simulink model "pto10Melo"  (R2021a)
settings: Solver=VariableStepAuto  StartTime=0.0  StopTime=10.0  RelTol=1e-3
values from neighbouring files (symbols this model uses):
  k = acker(A_aux, B_aux, p)    [Posibletaller3.m]
  L = acker(A', C', P1)'    [Posibletaller3.m]
undefined symbols (not defined in the file or in its folder): A, B, C
settings Model: Creator=User  LastModifiedBy=Cx001la
settings SolverCC: AlgebraicLoopSolver=TrustRegion
settings DebuggingCC: SFMachineParentedDataDiag=warning

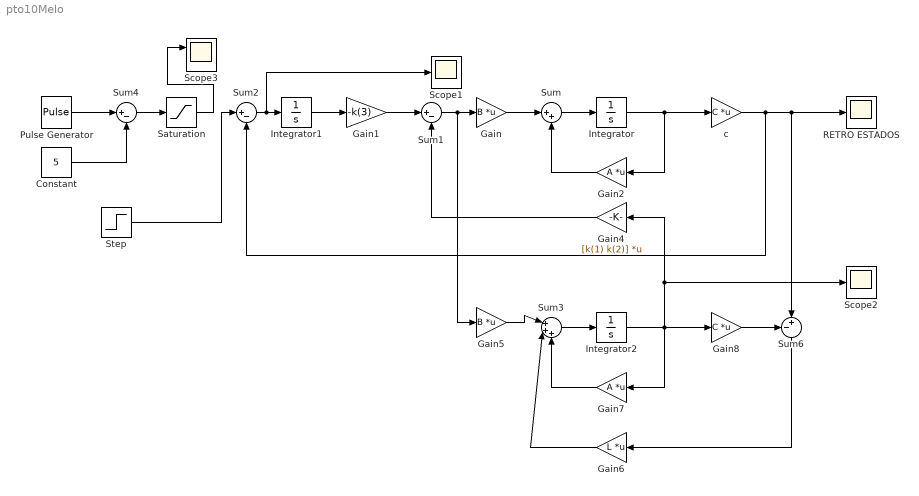
== system pto10Melo ==
  Constant : Constant  Value=5
  Gain : Gain  Gain=B  Multiplication=Matrix(K*u)
  Gain1 : Gain  Gain=-k(3)
  Gain2 : Gain  Gain=A  Multiplication=Matrix(K*u)
  Gain4 : Gain  Gain=[k(1) k(2)]  Multiplication=Matrix(K*u)
  Gain5 : Gain  Gain=B  Multiplication=Matrix(K*u)
  Gain6 : Gain  Gain=L  Multiplication=Matrix(K*u)
  Gain7 : Gain  Gain=A  Multiplication=Matrix(K*u)
  Gain8 : Gain  Gain=C  Multiplication=Matrix(K*u)
  Integrator : Integrator
  Integrator1 : Integrator
  Integrator2 : Integrator
  Pulse Generator : DiscretePulseGenerator  PulseType=Time based  Amplitude=10  Period=10  PulseWidth=50
  RETRO ESTADOS : Scope
  Saturation : Saturate  UpperLimit=3  LowerLimit=-3
  Scope1 : Scope
  Scope2 : Scope
  Scope3 : Scope  NumInputPorts=2
  Step : Step  Time=0  SampleTime=0
  Sum : Sum  Inputs=|++
  Sum1 : Sum  Inputs=|+-
  Sum2 : Sum  Inputs=|+-
  Sum3 : Sum  Inputs=|+++
  Sum4 : Sum  Inputs=|+-
  Sum6 : Sum  Inputs=-+|
  c : Gain  Gain=C  Multiplication=Matrix(K*u)
  wires:
  Gain/1 -> Sum/1
  Sum/1 -> Integrator/1
  Sum1/1 -> Gain5/1, Gain/1
  Gain2/1 -> Sum/2
  Integrator/1 -> c/1, Gain2/1
  Gain4/1 -> Sum1/2
  c/1 -> Sum6/2, RETRO ESTADOS/1, Sum2/2
  Gain1/1 -> Sum1/1
  Sum2/1 -> Scope1/1, Integrator1/1
  Integrator1/1 -> Gain1/1
  Integrator2/1 -> Scope2/1, Gain4/1, Gain7/1, Gain8/1
  Sum3/1 -> Integrator2/1
  Gain5/1 -> Sum3/1
  Gain8/1 -> Sum6/1
  Sum6/1 -> Gain6/1
  Gain7/1 -> Sum3/3
  Gain6/1 -> Sum3/2
  Saturation/1 -> Scope3/1
  Pulse Generator/1 -> Sum4/1
  Constant/1 -> Sum4/2
  Sum4/1 -> Saturation/1
  Step/1 -> Sum2/1
